simulink model "bumplessControl_CT"  (R2014b)
settings: Solver=ode45  StartTime=0.0  StopTime=10.0  RelTol=1e-3
settings Model: Creator=yujiang  LastModifiedBy=yujiang

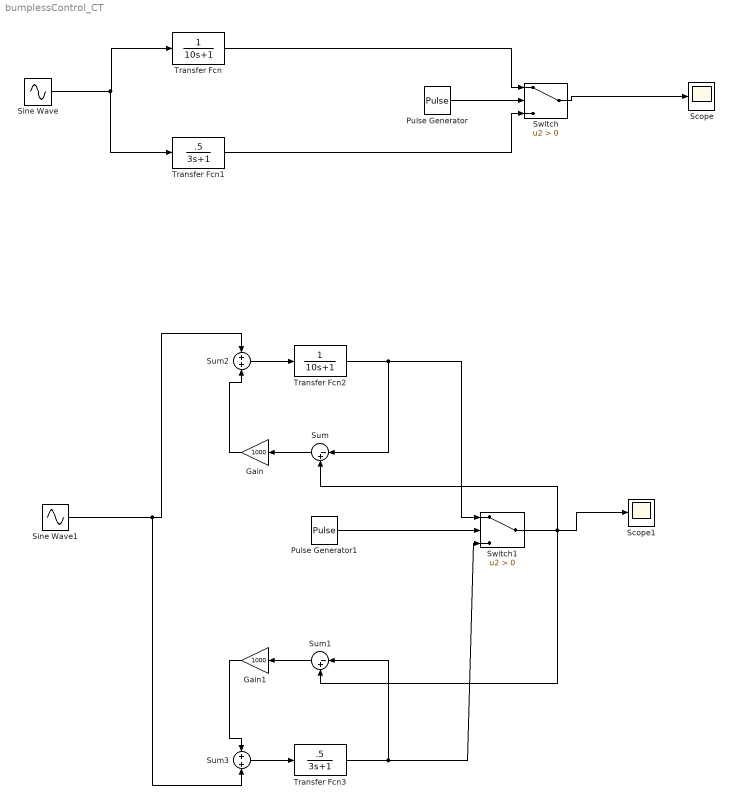
== system bumplessControl_CT ==
  Gain : Gain  Gain=1000
  Gain1 : Gain  Gain=1000
  Pulse Generator : DiscretePulseGenerator  PulseType=Time based  Period=1  PulseWidth=50
  Pulse Generator1 : DiscretePulseGenerator  PulseType=Time based  Period=1  PulseWidth=50
  Scope : Scope
  Scope1 : Scope
  Sine Wave : Sin  SampleTime=0.01
  Sine Wave1 : Sin  SampleTime=0.01
  Sum : Sum  Inputs=|-+
  Sum1 : Sum  Inputs=|-+
  Sum2 : Sum
  Sum3 : Sum
  Switch : Switch  Criteria=u2 > Threshold
  Switch1 : Switch  Criteria=u2 > Threshold
  Transfer Fcn : TransferFcn  Denominator=[10 1]
  Transfer Fcn1 : TransferFcn  Numerator=[.5]  Denominator=[3 1]
  Transfer Fcn2 : TransferFcn  Denominator=[10 1]
  Transfer Fcn3 : TransferFcn  Numerator=[.5]  Denominator=[3 1]
  wires:
  Sine Wave/1 -> Transfer Fcn1/1, Transfer Fcn/1
  Transfer Fcn/1 -> Switch/1
  Transfer Fcn1/1 -> Switch/3
  Pulse Generator/1 -> Switch/2
  Switch/1 -> Scope/1
  Sine Wave1/1 -> Sum3/2, Sum2/1
  Transfer Fcn2/1 -> Sum/1, Switch1/1
  Pulse Generator1/1 -> Switch1/2
  Sum/1 -> Gain/1
  Sum2/1 -> Transfer Fcn2/1
  Gain/1 -> Sum2/2
  Sum3/1 -> Transfer Fcn3/1
  Transfer Fcn3/1 -> Sum1/1, Switch1/3
  Switch1/1 -> Sum1/2, Sum/2, Scope1/1
  Sum1/1 -> Gain1/1
  Gain1/1 -> Sum3/1
